simulink model "BMS_Software_NXP"  (R2020a)
settings: Solver=FixedStepDiscrete  StartTime=0.0  StopTime=10.0  FixedStep=0.1  RelTol=1e-3
InitFcn:
  | mbd_s32k_consistency_checks(bdroot(gcs));
undefined symbols (not defined in the file or in its folder): CellTemp, CellVoltage, LQFP
libraries: mbd_s32k1xx_ec_toolbox x6, mbd_bcc_ec_toolbox x2, simulink x1
Description:
  | This model demonstrates how to use Model-Based Design Toolbox for S32K to run a BMS Algorithm, already validated in Matlab&Simulink environment.
  | This BMS Algorithm is available for free  on the Mathworks File Exchangehttps://www.mathworks.com/matlabcentral/fileexchange/72865-design-and-test-lithium-ion-battery-management-algorithms
  | 
  | Validation:
  | Hardware required: S32K144EVB + FRDM33772BSPIEVB + BATT-6EMULATOR
  | Once the model has been succesfully build it is automatically deployed on the target.
  | Open the BMS_Software_NXP.pmpx FreeMaster project, connect to the board and simulate the Algorithm states using the Cell Emulator.
settings Model: DataDictionary=BMS_Software_DD_NXP.sldd  EnableAccessToBaseWorkspace=off  PauseTimes=0  ExtModeTrigDuration=5  Creator=Chirag Patel  LastModifiedBy=rolan
settings SolverCC: AutoInsertRateTranBlk=on
settings DataIOCC: ExternalInput=off  InitialState=off  SaveOutput=off  SignalLogging=off  SaveTime=off
settings OptimizationCC: DefaultParameterBehavior=Inlined  EnhancedBackFolding=on  PassReuseOutputArgsAs=Individual arguments  ZeroExternalMemoryAtStartup=off  ZeroInternalMemoryAtStartup=off  OptimizeBlockOrder=speed  DifferentSizesBufferReuse=on  OptimizationCustomize=off  EfficientTunableParamExpr=on
settings DebuggingCC: UnderspecifiedInitializationDetection=Classic  MergeDetectMultiDrivingBlocksExec=none  InheritedTsInSrcMsg=none  SingleTaskRateTransMsg=error  ParameterTunabilityLossMsg=error  UnconnectedInputMsg=error  UnconnectedOutputMsg=error  UnconnectedLineMsg=error  UnknownTsInhSupMsg=error
settings HardwareCC: ProdBitPerPointer=32  ProdBitPerSizeT=32  ProdBitPerPtrDiffT=32  ProdLargestAtomicInteger=Long  ProdLargestAtomicFloat=Double  ProdWordSize=32  ProdHWDeviceType=ARM Compatible->ARM Cortex
settings ModelReferenceCC: ModelReferenceNumInstancesAllowed=Single  PropagateSignalLabelsOutOfModel=off
settings SFSimCC: MATLABDynamicMemAlloc=off
settings RTWCC: Description=Model Based Design Toolbox S32K1xx Code Generation Target  SystemTargetFile=mbd_s32k.tlc  MakeCommand=mbd_s32k_make_rtw COPY_MDLREF_INCLUDES=0  TemplateMakefile=mbd_s32k.tmf  GenerateReport=on  IncludeHyperlinkInReport=on  LaunchReport=on  GenerateTraceInfo=on  GenerateTraceReport=on  GenerateTraceReportSl=on  GenerateTraceReportSf=on  GenerateTraceReportEml=on
settings CodeAppCC: ForceParamTrailComments=on  IgnoreCustomStorageClasses=off  OperatorAnnotations=on  SimulinkDataObjDesc=on  SFDataObjDesc=on  InsertBlockDesc=on
settings STFCustomTargetCC: TargetLangStandard=C99 (ISO)  MultiwordLength=256  CombineOutputUpdateFcns=on  ERTCustomFileBanners=on  SupportContinuousTime=off  SupportNonInlinedSFcns=off  RemoveResetFunc=on  MATLABClassNameForMDSCustomization=Simulink.SoftwareTarget.ERTCustomization  SystemTargetFile=mbd_s32k.tlc
settings ERTTargetCC: TargetLangStandard=C99 (ISO)  ParMdlRefBuildCompliant=off  CompOptLevelCompliant=off  ConcurrentExecutionCompliant=off  ModelStepFunctionPrototypeControlCompliant=off  CPPClassGenCompliant=off  UseToolchainInfoCompliant=off  InlinedParameterPlacement=NonHierarchical  ERTSrcFileBannerTemplate=mbd_ert_code_template.cgt  ERTHdrFileBannerTemplate=mbd_ert_code_template.cgt  ERTDataSrcFileTemplate=mbd_ert_code_template.cgt  ERTDataHdrFileTemplate=mbd_ert_code_template.cgt  ERTCustomFileTemplate=example_file_process.tlc

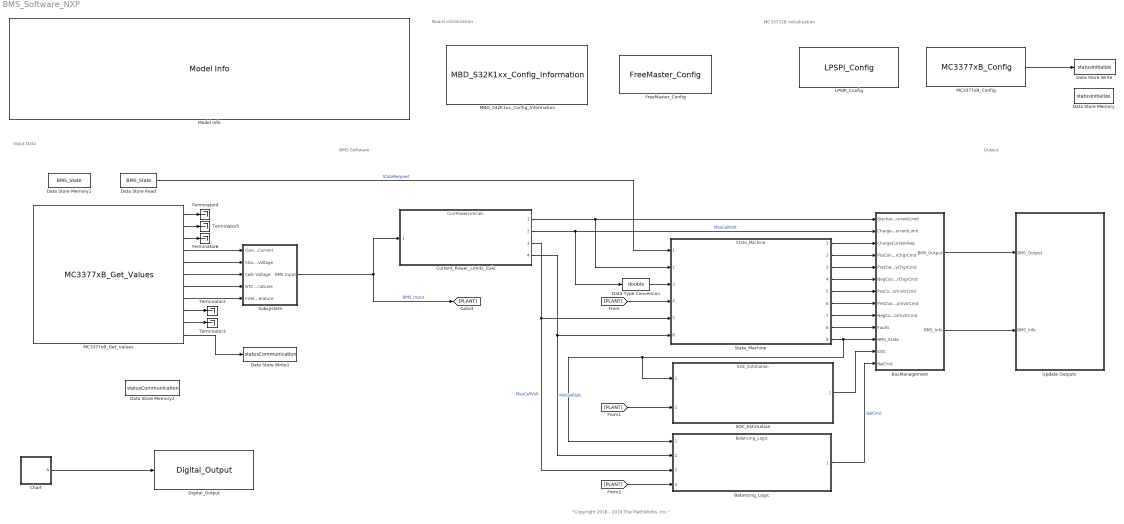
== system BMS_Software_NXP ==
  note: MC33772B initialization
  note: BMS Software
  note: "Copyright 2018 - 2019 The MathWorks, Inc."
  note: Board initialization
  note: Input Data
  note: Output
  Balancing_Logic : ModelReference  ModelNameDialog=Balancing_Logic  SimulationMode=Normal  ModelReferenceVersion=1.549
      mask Display: image('Balancing.jpg',[70,5,200,90])
  BusManagement : Subsystem
  Chart : Stateflow chart  TreatAsAtomicUnit=on
  Current_Power_Limits_Calc : ModelReference  ModelNameDialog=CurrPowerLimCalc.slx  SimulationMode=Normal  ModelReferenceVersion=1.534
      mask Display: image('CurrentPowerLimit.png',[68,15,80,80])
  Data Store Memory : DataStoreMemory  DataStoreName=statusInitialize  ReadBeforeWriteMsg=warning  WriteAfterWriteMsg=warning  WriteAfterReadMsg=warning  ShowAdditionalParam=off
  Data Store Memory1 : DataStoreMemory  DataStoreName=BMS_State  ReadBeforeWriteMsg=warning  WriteAfterWriteMsg=warning  WriteAfterReadMsg=warning  InitialValue=SRE.Driving  ShowAdditionalParam=off  OutDataTypeStr=Enum: SRE
  Data Store Memory2 : DataStoreMemory  DataStoreName=statusCommunication  ReadBeforeWriteMsg=warning  WriteAfterWriteMsg=warning  WriteAfterReadMsg=warning  ShowAdditionalParam=off
  Data Store Read : DataStoreRead  DataStoreName=BMS_State
  Data Store Write : DataStoreWrite  DataStoreName=statusInitialize
  Data Store Write1 : DataStoreWrite  DataStoreName=statusCommunication
  Data Type Conversion : DataTypeConversion  OutDataTypeStr=double
  Digital_Output : mbd_s32k1xx_ec_toolbox/GPIO Blocks/Digital_Output  gpio_pin=PTD0: [PTD0 | Port D I/O]  init_val=Low  drive_strength=Low
  FreeMaster_Config : mbd_s32k1xx_ec_toolbox/Utility Blocks/FreeMaster_Config  interface=LPUART1  baudrate=115200  rxd=PTC6: [LPUART1_RX | Receive]  txd=PTC7: [LPUART1_TX | Transmit]  mode=Short Interrupt  isr_prio=1  show_adv_opts=on  use_scope=on  max_scope_vars=8  use_recorder=off  max_rec_vars=8  rec_buff_size=1024  rec_timebase=0 milliseconds  comm_buffer_size_auto=on  comm_buffer_size=255  comm_rqueue_size_default=on  comm_rqueue_size=32
  "LPSPI_Config " : mbd_s32k1xx_ec_toolbox/Communication Blocks/SPI Blocks/LPSPI_Config   InstanceNumber=0  Role=Master  BaudRate=1000000  ShowAdvanced=on  sin=PTB3: [LPSPI0_SIN | LPSPI Serial Data Input]  sout=PTB4: [LPSPI0_SOUT | LPSPI Serial Data Output]  sck=PTB2: [LPSPI0_SCK | LPSPI Serial Clock I/O]  pcs0=None  pcs1=PTB5: [LPSPI0_PCS1 | Peripheral Chip Select 1]  pcs2=None  pcs3=None  CPHA=1  CPOL=0  BitOrder=MSB first  TransferSize=40  WhichPCS=0  PCSPol=ActiveLow  ContinuousTransfer=off
  MBD_S32K1xx_Config_Information : mbd_s32k1xx_ec_toolbox/MBD_S32K1xx_Config_Information  mbdt_ver=0  disp_str=|  config_params=[]  mcu_target_name=S32K144  mcu_target_package=100-LQFP  mcu_target_sram_size=64KB  mcu_system_clock_freq=80  mcu_xtal_freq=External 8  mcu_steptick_timer=LPIT Channel 0  mcu_steptick_prio=15  ds_import_enable=on  target_compiler=GCC  target_memory=FLASH  gcc_target_compile_opts=-mthumb -mfloat-abi=hard -mfpu=fpv4-sp-d16 -O1 -g -gstrict-dwarf  gcc_target_assemble_opts=-mthumb -mfloat-abi=hard -mfpu=fpv4-sp-d16 -g  gcc_target_link_opts=-mthumb -mfloat-abi=hard -mfpu=fpv4-sp-d16  gcc_target_default_lcf=on  gcc_target_user_lcf=S32K148_192_flash.ld  ghs_target_compile_opts=-cpu=cortexm4f -thumb -fpu=vfpv4_d16 -fsingle -Ogeneral -Wundef -Wimplicit-int -Wshadow -Wtrigraphs --no_commons --gnu_asm -gnu99 -gdwarf-2 -G  ghs_target_assemble_opts=-cpu=cortexm4f -fpu=vfpv4_d16  ghs_target_link_opts=-cpu=cortexm4f -thumb -fpu=vfpv4_d16  ghs_target_default_lcf=on  ghs_target_user_lcf=S32K148_192_flash.ld  iar_target_compile_opts=--cpu=Cortex-M4F --thumb --fpu=VFPv4_sp -Ol -e --debug --dlib_config normal  iar_target_assemble_opts=--cpu Cortex-M4F --thumb --fpu VFPv4_sp  iar_target_link_opts=--no_exceptions --vfe --inline  iar_target_default_lcf=on  iar_target_user_lcf=S32K148_192_flash.icf  pil_download_enable=off  rbl_download_enable=on  rbl_start_delay=5000  rbl_download_interface=OpenSDA  rbl_restart_request=off  rbl_com_port=Custom  rbl_com_port_custom=COM1  pil_download_rate=57600  pil_opensda_drive=Custom  pil_opensda_drive_custom=D  pil_uart_instance=1  pil_uart_rx=PTC6: [LPUART1_RX | Receive]  pil_uart_tx=PTC7: [LPUART1_TX | Transmit]  FTM_PWM_PcrCheckEnDis=on  FTM_Input_Edge_Inputs_PcrCheckEnDis=on  FTM_Dual_Edge_Inputs_PcrCheckEnDis=on  FTM_Quadrature_Inputs_PcrCheckEnDis=on  FTM_Hall_Sensor_Inputs_PcrCheckEnDis=on  LPTMR_PcrCheckEnDis=on  PIT_PcrCheckEnDis=on  RTC_PcrCheckEnDis=on  FlexCAN_PcrCheckEnDis=on  LIN_PcrCheckEnDis=on  FlexIO_PcrCheckEnDis=on  LPI2C_PcrCheckEnDis=on  LPSPI_PcrCheckEnDis=on  LPUART_PcrCheckEnDis=on  CMP_PcrCheckEnDis=on  GPIO_OutputPcrCheckEnDis=on  GPIO_InputPcrCheckEnDis=on  SBC_PcrCheckEnDis=on  BMS_PcrCheckEnDis=on  AMMCLIB_PcrCheckEnDis=on  FM_PcrCheckEnDis=on  Profile_PcrCheckEnDis=on  ConfigParams_PcrCheckEnDis=on  ModelRef_PcrCheckEnDis=on  PDB0_PcrCheckEnDis=on  CSEc_PcrCheckEnDis=on  eDMA_PcrCheckEnDis=on  FLASH_PcrCheckEnDis=on  ADC_PcrCheckEnDis=on  WDOG_PcrCheckEnDis=on
      | Target : S32K144-64KB_SRAM
      | Package : 100-pin
      | System clock : 80 MHz
      | XTAL clock : External 8 MHz
      | Compiler : IAR
      | Target Type : FLASH
      | Download Code after build : off
      | Step Tick Interrupt Priority : 15
  MC3377xB_Config : mbd_bcc_ec_toolbox/BMS/MC3377xB_Config  Priority=1  bccInstance=0  bccMode=SPI  bccTPLDevNr=1  bccSpiDev=MC33772B  bccSpiCell=6  bccTPLDev1=MC33771B  bccTPLCell1=3  bccTPLDev2=MC33771B  bccTPLCell2=3  bccTPLDev3=MC33771B  bccTPLCell3=3  bccTPLDev4=MC33771B  bccTPLCell4=3  bccTPLDev5=MC33771B  bccTPLCell5=3  bccTPLDev6=MC33771B  bccTPLCell6=3  bccTPLDev7=MC33771B  bccTPLCell7=3  bccTPLDev8=MC33771B  bccTPLCell8=3  bccTPLDev9=MC33771B  bccTPLCell9=3  bccTPLDev10=MC33771B  bccTPLCell10=3  bccTPLDev11=MC33771B  bccTPLCell11=3  bccTPLDev12=MC33771B  bccTPLCell12=3  bccTPLDev13=MC33771B  bccTPLCell13=3  bccTPLDev14=MC33771B  bccTPLCell14=3  bccTPLDev15=MC33771B  bccTPLCell15=3  bccSpiMaster=0  bccSPIMasterCSCustom=on  bccSPIMasterPCS=LPSPI_PCS1  bccSPIMasterPCSGPIO=PTA0: [PTA0 | Port A I/O]  bccSpiSlave=0  bccSPISlavePCS=LPSPI_PCS1  bccSPI_RESET_ALT0=PTD4: [PTD4 | Port D I/O]  bccTPL_ENABLE=PTA0: [PTA0 | Port A I/O]  bccTPL_INTB=PTA0: [PTA0 | Port A I/O]  bccNTCBeta=3900  bccNTCRes=6800  bccNTCRefR=10000  bccNTCRefT=25  bccShunt=100000
  MC3377xB_Get_Values : mbd_bcc_ec_toolbox/BMS/MC3377xB_Get_Values  bccInstance=0  bccCid=1  bccStartConversion=on
  Model Info : simulink/Model-Wide Utilities/Model Info  Frame=off  DisplayStringWithTags=|  HorizontalTextAlignment=Left  LeftAlignmentValue=0.02
      | Model Name: %<ModelName>
      | 
      | Description: %<Description>
  SOC_Estimation : ModelReference  ModelNameDialog=SOC_Estimation.slx  SimulationMode=Normal  ModelReferenceVersion=1.763
      mask Display: image('SOC.jpg',[100,15,150,75])
  State_Machine : ModelReference  ModelNameDialog=State_Machine  SimulationMode=Normal  ModelReferenceVersion=1.672
      mask Display: image('StateMachine.jpg',[80,40,130,130])
  Subsystem : Subsystem
  Terminator{2..6} (5 alike) : Terminator
  Update Outputs : Subsystem
  wires:
  State_Machine/9 -> SOC_Estimation/1, Balancing_Logic/1, BusManagement/11(BMS_State)
  Data Store Read/1 -> State_Machine/1  "StateRequest"
  Current_Power_Limits_Calc/3 -> State_Machine/5, Balancing_Logic/3  "MaxCellVolt"
  Current_Power_Limits_Calc/4 -> Balancing_Logic/2, State_Machine/6  "MinCellVolt"
  [PLANT] -> Balancing_Logic/4
  [PLANT] -> State_Machine/4
  [PLANT] -> SOC_Estimation/2
  State_Machine/1 -> BusManagement/3(ChargeCurrentReq)
  State_Machine/2 -> BusManagement/4(PosContactorChgrCmd)
  State_Machine/3 -> BusManagement/5(PreChargeRelayChgrCmd)
  State_Machine/4 -> BusManagement/6(NegContactorChgrCmd)
  State_Machine/5 -> BusManagement/7(PosContactorInvtrCmd)
  State_Machine/6 -> BusManagement/8(PreChargeRelayInvtrCmd)
  State_Machine/7 -> BusManagement/9(NegContactorInvtrCmd)
  State_Machine/8 -> BusManagement/10(Faults)
  SOC_Estimation/1 -> BusManagement/12(SOC)
  Balancing_Logic/1 -> BusManagement/13(BalCmd)  "BalCmd"
  BusManagement/1(BMS_Output) -> Update Outputs/1(BMS_Output)
  BusManagement/2(BMS_Info) -> Update Outputs/2(BMS_Info)
  Current_Power_Limits_Calc/1 -> BusManagement/1(DischargeCurrentLimit), State_Machine/2
  Current_Power_Limits_Calc/2 -> Data Type Conversion/1, BusManagement/2(ChargeCurrentLimit)  "MaxCellVolt"
  MC3377xB_Get_Values/6 -> Subsystem/3(Cells Voltage)
  MC3377xB_Get_Values/2 -> Terminator5/1
  MC3377xB_Get_Values/5 -> Subsystem/2(Stack Voltage)
  MC3377xB_Get_Values/11 -> Data Store Write1/1
  MC3377xB_Get_Values/7 -> Subsystem/4(NTC Temperatures)
  Subsystem/1(BMS Input) -> Current_Power_Limits_Calc/1, [PLANT]  "BMS_Input"
  MC3377xB_Get_Values/1 -> Terminator4/1
  MC3377xB_Get_Values/3 -> Terminator6/1
  MC3377xB_Get_Values/4 -> Subsystem/1(ISense Current)
  MC3377xB_Get_Values/10 -> Terminator3/1
  MC3377xB_Get_Values/8 -> Subsystem/5(Internal Temperature)
  MC3377xB_Get_Values/9 -> Terminator2/1
  MC3377xB_Config/1 -> Data Store Write/1
  Data Type Conversion/1 -> State_Machine/3
  Chart/1(" A") -> Digital_Output/1

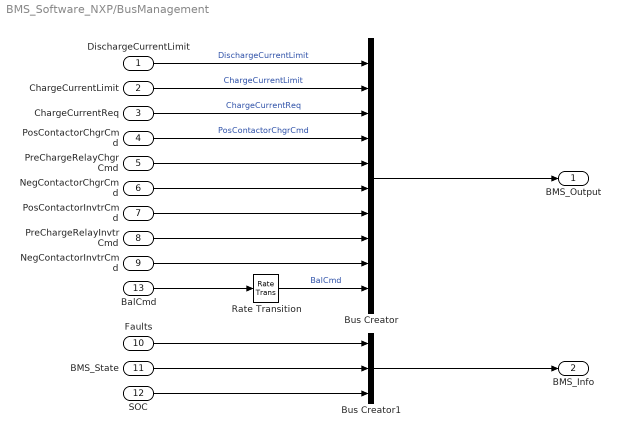
== system BMS_Software_NXP/BusManagement ==
  DischargeCurrentLimit : Inport
  ChargeCurrentLimit : Inport  Port=2
  ChargeCurrentReq : Inport  Port=3
  PosContactorChgrCmd : Inport  Port=4
  PreChargeRelayChgrCmd : Inport  Port=5
  NegContactorChgrCmd : Inport  Port=6
  PosContactorInvtrCmd : Inport  Port=7
  PreChargeRelayInvtrCmd : Inport  Port=8
  NegContactorInvtrCmd : Inport  Port=9
  Faults : Inport  Port=10
  BMS_State : Inport  Port=11
  SOC : Inport  Port=12
  BalCmd : Inport  Port=13
  Bus Creator1 : BusCreator  Inputs=3  OutDataTypeStr=Bus: BMS_Info  NonVirtualBus=on
  Bus Creator : BusCreator  Inputs=10  OutDataTypeStr=Bus: BMS_Output  NonVirtualBus=on
  Rate Transition : RateTransition  Integrity=off  Deterministic=off
  BMS_Output : Outport
  BMS_Info : Outport  Port=2  OutDataTypeStr=Bus: BMS_Info
  wires:
  PosContactorInvtrCmd/1 -> Bus Creator/7
  PreChargeRelayChgrCmd/1 -> Bus Creator/5
  PosContactorChgrCmd/1 -> Bus Creator/4  "PosContactorChgrCmd"
  NegContactorInvtrCmd/1 -> Bus Creator/9
  Faults/1 -> Bus Creator1/1
  NegContactorChgrCmd/1 -> Bus Creator/6
  PreChargeRelayInvtrCmd/1 -> Bus Creator/8
  Bus Creator1/1 -> BMS_Info/1
  BalCmd/1 -> Rate Transition/1
  Bus Creator/1 -> BMS_Output/1
  SOC/1 -> Bus Creator1/3
  BMS_State/1 -> Bus Creator1/2
  ChargeCurrentLimit/1 -> Bus Creator/2  "ChargeCurrentLimit"
  DischargeCurrentLimit/1 -> Bus Creator/1  "DischargeCurrentLimit"
  ChargeCurrentReq/1 -> Bus Creator/3  "ChargeCurrentReq"
  Rate Transition/1 -> Bus Creator/10  "BalCmd"

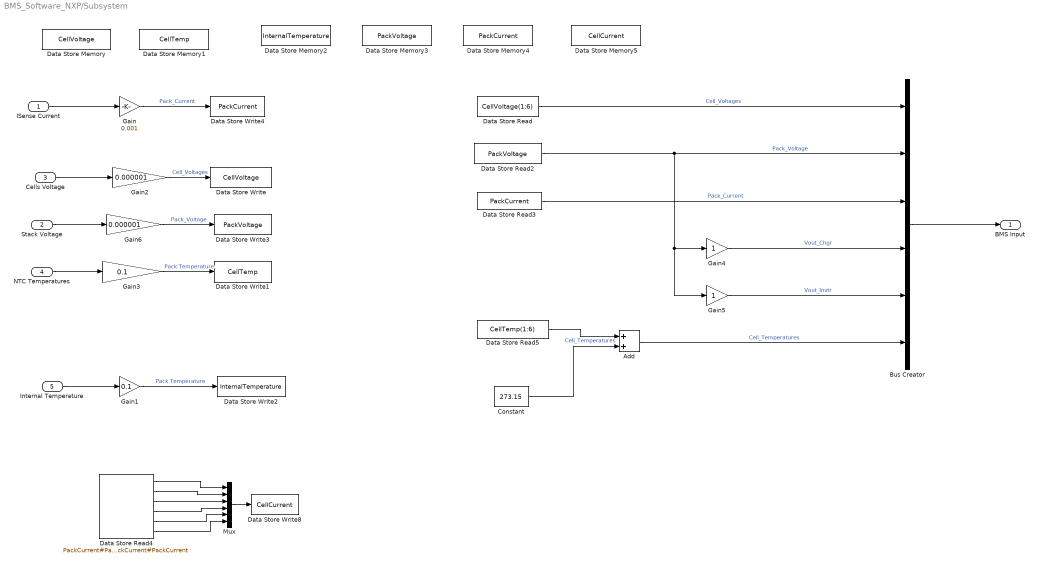
== system BMS_Software_NXP/Subsystem ==
  ISense Current : Inport
  Stack Voltage : Inport  Port=2
  Cells Voltage : Inport  Port=3
  NTC Temperatures : Inport  Port=4
  Internal Temperature : Inport  Port=5
  Add : Sum  AccumDataTypeStr=single
  Bus Creator : BusCreator  Inputs=6  OutDataTypeStr=Bus: BMS_Input  NonVirtualBus=on
  Constant : Constant  Value=273.15  OutDataTypeStr=single
  Data Store Memory : DataStoreMemory  DataStoreName=CellVoltage  ReadBeforeWriteMsg=warning  WriteAfterWriteMsg=warning  WriteAfterReadMsg=warning  InitialValue=zeros(1,14)  ShowAdditionalParam=off  OutDataTypeStr=single
  Data Store Memory1 : DataStoreMemory  DataStoreName=CellTemp  ReadBeforeWriteMsg=warning  WriteAfterWriteMsg=warning  WriteAfterReadMsg=warning  InitialValue=zeros(1,7)  ShowAdditionalParam=off  OutDataTypeStr=single
  Data Store Memory2 : DataStoreMemory  DataStoreName=InternalTemperature  ReadBeforeWriteMsg=warning  WriteAfterWriteMsg=warning  WriteAfterReadMsg=warning  ShowAdditionalParam=off  OutDataTypeStr=single
  Data Store Memory3 : DataStoreMemory  DataStoreName=PackVoltage  ReadBeforeWriteMsg=warning  WriteAfterWriteMsg=warning  WriteAfterReadMsg=warning  ShowAdditionalParam=off  OutDataTypeStr=single
  Data Store Memory4 : DataStoreMemory  DataStoreName=PackCurrent  ReadBeforeWriteMsg=warning  WriteAfterWriteMsg=warning  WriteAfterReadMsg=warning  ShowAdditionalParam=off  OutDataTypeStr=single
  Data Store Memory5 : DataStoreMemory  DataStoreName=CellCurrent  ReadBeforeWriteMsg=warning  WriteAfterWriteMsg=warning  WriteAfterReadMsg=warning  InitialValue=zeros(1,6) + 300  ShowAdditionalParam=off  OutDataTypeStr=single
  Data Store Read : DataStoreRead  DataStoreName=CellVoltage  DataStoreElements=CellVoltage(1:6)
  Data Store Read2 : DataStoreRead  DataStoreName=PackVoltage
  Data Store Read3 : DataStoreRead  DataStoreName=PackCurrent
  Data Store Read4 : DataStoreRead  DataStoreName=PackCurrent  DataStoreElements=PackCurrent#PackCurrent#PackCurrent#PackCurrent#PackCurrent#PackCurrent
  Data Store Read5 : DataStoreRead  DataStoreName=CellTemp  DataStoreElements=CellTemp(1:6)
  Data Store Write : DataStoreWrite  DataStoreName=CellVoltage
  Data Store Write1 : DataStoreWrite  DataStoreName=CellTemp
  Data Store Write2 : DataStoreWrite  DataStoreName=InternalTemperature
  Data Store Write3 : DataStoreWrite  DataStoreName=PackVoltage
  Data Store Write4 : DataStoreWrite  DataStoreName=PackCurrent
  Data Store Write8 : DataStoreWrite  DataStoreName=CellCurrent
  Gain : Gain  Gain=0.001  OutDataTypeStr=single
  Gain1 : Gain  Gain=0.1  OutDataTypeStr=single
  Gain2 : Gain  Gain=0.000001  OutDataTypeStr=single
  Gain3 : Gain  Gain=0.1  OutDataTypeStr=single
  Gain4 : Gain  OutDataTypeStr=single
  Gain5 : Gain  OutDataTypeStr=single
  Gain6 : Gain  Gain=0.000001  OutDataTypeStr=single
  Mux : Mux  Inputs=6
  BMS Input : Outport
  wires:
  Data Store Read2/1 -> Gain5/1, Gain4/1, Bus Creator/2  "Pack_Voltage"
  ISense Current/1 -> Gain/1
  Bus Creator/1 -> BMS Input/1
  Constant/1 -> Add/2
  Gain4/1 -> Bus Creator/4  "Vout_Chgr"
  Gain5/1 -> Bus Creator/5  "Vout_Invtr"
  Data Store Read/1 -> Bus Creator/1  "Cell_Voltages"
  Cells Voltage/1 -> Gain2/1
  NTC Temperatures/1 -> Gain3/1
  Gain2/1 -> Data Store Write/1  "Cell_Voltages"
  Internal Temperature/1 -> Gain1/1
  Stack Voltage/1 -> Gain6/1
  Gain6/1 -> Data Store Write3/1  "Pack_Voltage"
  Gain/1 -> Data Store Write4/1  "Pack_Current"
  Data Store Read3/1 -> Bus Creator/3  "Pack_Current"
  Gain1/1 -> Data Store Write2/1  "Pack Temperature"
  Data Store Read4/6 -> Mux/6
  Mux/1 -> Data Store Write8/1
  Data Store Read4/4 -> Mux/4
  Data Store Read4/5 -> Mux/5
  Data Store Read4/2 -> Mux/2
  Data Store Read4/3 -> Mux/3
  Data Store Read4/1 -> Mux/1
  Data Store Read5/1 -> Add/1  "Cell_Temperatures"
  Gain3/1 -> Data Store Write1/1  "Pack Temperature"
  Add/1 -> Bus Creator/6  "Cell_Temperatures"

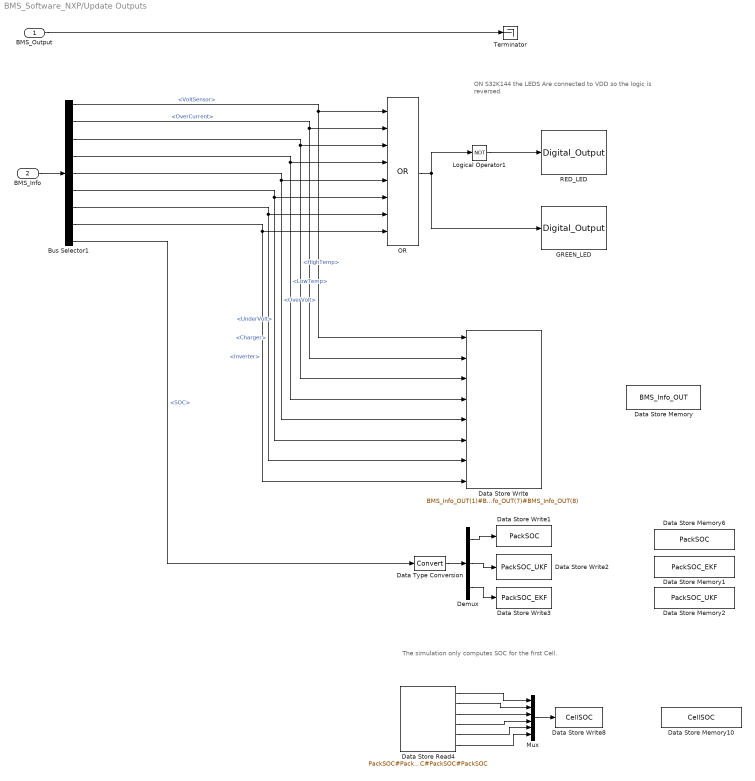
== system BMS_Software_NXP/Update Outputs ==
  note: ON S32K144 the LEDS Are connected to VDD so the logic is reversed.
  note: The simulation only computes SOC for the first Cell.
  BMS_Output : Inport
  BMS_Info : Inport  Port=2
  Bus Selector1 : BusSelector  OutputSignals=Faults.VoltSensor,Faults.OverCurrent,Faults.HighTemp,Faults.LowTemp,Faults.OverVolt,Faults.UnderVolt,Faults.Charger,Faults.Inverter,SOC
  Data Store Memory : DataStoreMemory  DataStoreName=BMS_Info_OUT  ReadBeforeWriteMsg=warning  WriteAfterWriteMsg=warning  WriteAfterReadMsg=warning  InitialValue=[0 0 0 0 0 0 0 0]  ShowAdditionalParam=off  OutDataTypeStr=boolean
  Data Store Memory1 : DataStoreMemory  DataStoreName=PackSOC_EKF  ReadBeforeWriteMsg=warning  WriteAfterWriteMsg=warning  WriteAfterReadMsg=warning  ShowAdditionalParam=off  OutDataTypeStr=single
  Data Store Memory10 : DataStoreMemory  DataStoreName=CellSOC  ReadBeforeWriteMsg=warning  WriteAfterWriteMsg=warning  WriteAfterReadMsg=warning  InitialValue=zeros(1,6)  ShowAdditionalParam=off  OutDataTypeStr=single
  Data Store Memory2 : DataStoreMemory  DataStoreName=PackSOC_UKF  ReadBeforeWriteMsg=warning  WriteAfterWriteMsg=warning  WriteAfterReadMsg=warning  ShowAdditionalParam=off  OutDataTypeStr=single
  Data Store Memory6 : DataStoreMemory  DataStoreName=PackSOC  ReadBeforeWriteMsg=warning  WriteAfterWriteMsg=warning  WriteAfterReadMsg=warning  ShowAdditionalParam=off  OutDataTypeStr=single
  Data Store Read4 : DataStoreRead  DataStoreName=PackSOC  DataStoreElements=PackSOC#PackSOC#PackSOC#PackSOC#PackSOC#PackSOC
  Data Store Write : DataStoreWrite  DataStoreName=BMS_Info_OUT  DataStoreElements=BMS_Info_OUT(1)#BMS_Info_OUT(2)#BMS_Info_OUT(3)#BMS_Info_OUT(4)#BMS_Info_OUT(5)#BMS_Info_OUT(6)#BMS_Info_OUT(7)#BMS_Info_OUT(8)
  Data Store Write1 : DataStoreWrite  DataStoreName=PackSOC
  Data Store Write2 : DataStoreWrite  DataStoreName=PackSOC_UKF
  Data Store Write3 : DataStoreWrite  DataStoreName=PackSOC_EKF
  Data Store Write8 : DataStoreWrite  DataStoreName=CellSOC
  Data Type Conversion : DataTypeConversion
  Demux : Demux  Outputs=3
  GREEN_LED : mbd_s32k1xx_ec_toolbox/GPIO Blocks/Digital_Output  gpio_pin=PTD16: [PTD16 | Port D I/O]  init_val=Low  drive_strength=Low
  Logical Operator1 : Logic  Operator=NOT  AllPortsSameDT=off  OutDataTypeStr=boolean
  Mux : Mux  Inputs=6
  OR : Logic  Operator=OR  Inputs=8  AllPortsSameDT=off  OutDataTypeStr=boolean
  RED_LED : mbd_s32k1xx_ec_toolbox/GPIO Blocks/Digital_Output  gpio_pin=PTD15: [PTD15 | Port D I/O]  init_val=Low  drive_strength=Low
  Terminator : Terminator
  wires:
  Bus Selector1/4 -> OR/4, Data Store Write/4  "<LowTemp>"
  Bus Selector1/8 -> Data Store Write/8, OR/8  "<Inverter>"
  OR/1 -> GREEN_LED/1, Logical Operator1/1
  Bus Selector1/5 -> Data Store Write/5, OR/5  "<OverVolt>"
  Bus Selector1/7 -> Data Store Write/7, OR/7  "<Charger>"
  Bus Selector1/3 -> Data Store Write/3, OR/3  "<HighTemp>"
  Bus Selector1/1 -> Data Store Write/1, OR/1  "<VoltSensor>"
  Bus Selector1/6 -> Data Store Write/6, OR/6  "<UnderVolt>"
  Bus Selector1/2 -> Data Store Write/2, OR/2  "<OverCurrent>"
  BMS_Info/1 -> Bus Selector1/1
  BMS_Output/1 -> Terminator/1
  Logical Operator1/1 -> RED_LED/1
  Bus Selector1/9 -> Data Type Conversion/1  "<SOC>"
  Data Type Conversion/1 -> Demux/1
  Demux/1 -> Data Store Write1/1
  Demux/2 -> Data Store Write2/1
  Demux/3 -> Data Store Write3/1
  Data Store Read4/5 -> Mux/5
  Data Store Read4/3 -> Mux/3
  Mux/1 -> Data Store Write8/1
  Data Store Read4/4 -> Mux/4
  Data Store Read4/2 -> Mux/2
  Data Store Read4/1 -> Mux/1
  Data Store Read4/6 -> Mux/6

== stateflow chart BMS_Software_NXP/Chart ==
  state A
  state A1
  (default) -> A
  A -> A1
  A1 -> A
  data: A output boolean [0..1]
